simulink model "c2407adcpwmtest"  (Simulink 6.0)
settings: Solver=FixedStepDiscrete  StartTime=0.0  StopTime=inf  RelTol=1e-3
libraries: c2400dspchiplib x2, c2000tgtpreflib x1
settings Model: Creator=zgalijas  LastModifiedBy=zgalijas  ProdHWDeviceType=TI C2000
settings DataIOCC: SaveOutput=off  SaveTime=off  SignalLoggingName=logsOut
settings OptimizationCC: InlineInvariantSignals=off
settings DebuggingCC: CheckExecutionContextPreStartOutputMsg=on  CheckExecutionContextRuntimeOutputMsg=on  SolverPrmCheckMsg=none
settings HardwareCC: ProdBitPerChar=16  ProdBitPerInt=16  ProdIntDivRoundTo=Zero  ProdEndianess=LittleEndian  ProdWordSize=16  ProdHWDeviceType=TI C2000  TargetHWDeviceType=32-bit Generic
settings ModelReferenceCC: UpdateModelReferenceTargets=IfOutOfDate
settings RTWCC: SystemTargetFile=ti_c2000_grt.tlc  GenCodeOnly=on  TemplateMakefile=ti_c2000_grt.tmf  ProcessScript=ti_c2000_grt_make_rtw_hook
settings STFCustomTargetCC: TargetFcnLib=ansi_tfl_tmw.mat  GenFloatMathFcnCalls=ANSI_C  ModelReferenceCompliant=off  SystemTargetFile=ti_c2000_grt.tlc  ActivateCallback=ti_c2000_callback('ActivateCallback',hSrc,hDlg);  ForcedBaseTarget=off
settings GRTTargetCC: ModelReferenceCompliant=off  MatFileLogging=off
settings SFSimCC: SFSimApplyToAllLibs=on  SFSimBuildMode=Incremental

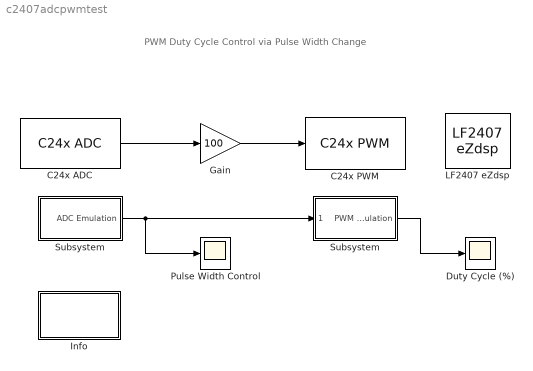
== system c2407adcpwmtest ==
  note: PWM Duty Cycle Control via Pulse Width Change
  " Info" : Subsystem  PropExecContextAcrossSSBoundary=on
      mask Display: disp('Info')
  C24x ADC : c2400dspchiplib/C24x ADC  useModule=A  A0=on  A1=off  A2=off  A3=off  A4=off  A5=off  A6=off  A7=off  B0=on  B1=off  B2=off  B3=off  B4=off  B5=off  B6=off  B7=off  sampleTime=64/80000  sourceSOC=Software
  C24x PWM : c2400dspchiplib/C24x PWM  useModule=A  timerSource=Specify via dialog  timerPeriod=64000  waveformType=Asymmetric  unit1Status=on  unit1Source=Input port  unit1Value=2000  unit2Status=off  unit2Source=Input port  unit2Value=2000  unit3Status=off  unit3Source=Input port  unit3Value=2000  unit1_1Logic=Active high  unit1_2Logic=Active low  unit2_1Logic=Active high  unit2_2Logic=Active low  unit3_1Logic=Active high  unit3_2Logic=Active low  enableDeadband1=on  enableDeadband2=off  enableDeadband3=off  deadbandPrescaler=16  deadbandPeriod=12  adcstartEvent=None
  Duty Cycle (%) : Scope
      settings: YMin=10  YMax=90
  Gain : Gain  Gain=100  ParameterScaling=2^-15  OutDataTypeMode=Specify via dialog  OutDataType=uint(16)  OutScaling=2^-10
  LF2407 eZdsp : c2000tgtpreflib/LF2407 eZdsp  Tag=C2000 TARGET PREFERENCES BLOCK
  Pulse Width Control : Scope
      settings: YMin=0.2  YMax=1.4
  Subsystem : Subsystem  PropExecContextAcrossSSBoundary=on
  "Subsystem " : Subsystem  Tag=sdfsfsf  PropExecContextAcrossSSBoundary=on
  wires:
  C24x ADC/1 -> Gain/1
  "Subsystem "/1(ADC Emulation) -> Pulse Width Control/1, Subsystem/1(" ")
  Gain/1 -> C24x PWM/1
  Subsystem/1(PWM Emulation) -> Duty Cycle (%)/1

== system c2407adcpwmtest/ Info ==
  note: Demo Description:
  note: Setup:
  note: The code generation portion of this demo requires the following hardware:
      |
      | Spectrum Digital eZdsp LF2407
      | Function generator
      | Oscilloscope and probes
      |
      | Connect the function generator output to the ADC input ADCINA0 on the eZdsp LF2407.
      | Connect the output of PWM1 on the eZdsp LF2407 to the analog input of the oscilloscope.
  note: This example demonstrates the use of the c24x ADC block to sample an analog voltage
      | and the c24x PWM block to generate a pulse waveform. The analog voltage controls the
      | duty cycle of the PWM. Duty cycle change can be observed on the oscilloscope.
      |
      | For results of generated code to match the simulation, apply a pulse waveform toggling
      | between 0.5 and 1.5 V every 2 s.

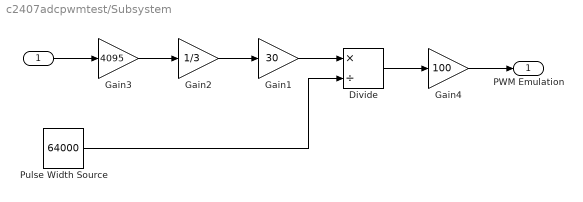
== system c2407adcpwmtest/Subsystem ==
  " " : Inport  LatchInput=off
  Divide : Product  Inputs=*/  OutScaling=2^-10
  Gain1 : Gain  Gain=30  ParameterScaling=2^-15  OutDataType=uint(16)  OutScaling=2^-10
  Gain2 : Gain  Gain=1/3  ParameterScaling=2^-15  OutDataType=uint(16)  OutScaling=2^-10
  Gain3 : Gain  Gain=4095  ParameterScaling=2^-15  OutDataType=uint(16)  OutScaling=2^-10
  Gain4 : Gain  Gain=100  ParameterScaling=2^-15  OutDataType=uint(16)  OutScaling=2^-10
  Pulse Width Source : Constant  Value=64000  OutDataTypeMode=single  ConRadixGroup=Best Precision: Vector-wise  OutScaling=2^-10
  PWM Emulation : Outport
  wires:
  Gain3/1 -> Gain2/1
  Gain2/1 -> Gain1/1
  " "/1 -> Gain3/1
  Gain1/1 -> Divide/1
  Divide/1 -> Gain4/1
  Pulse Width Source/1 -> Divide/2
  Gain4/1 -> PWM Emulation/1

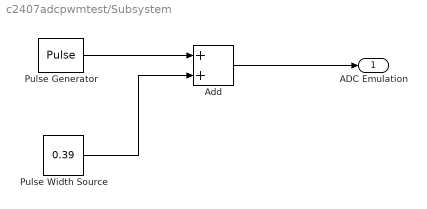
== system c2407adcpwmtest/Subsystem  ==
  Add : Sum  OutScaling=2^-10
  Pulse Generator : DiscretePulseGenerator  Amplitude=0.78  Period=4000  PulseWidth=2000  SampleTime=64/80000
  Pulse Width Source : Constant  Value=0.39  OutDataTypeMode=single  ConRadixGroup=Best Precision: Vector-wise  OutScaling=2^-10
  ADC Emulation : Outport
  wires:
  Pulse Generator/1 -> Add/1
  Pulse Width Source/1 -> Add/2
  Add/1 -> ADC Emulation/1
